simulink model "Matlab_ReadUART"  (R2022b)
settings: Solver=FixedStepAuto  StartTime=0.0  StopTime=inf  FixedStep=0.02  RelTol=1e-3
undefined symbols (not defined in the file): LF
libraries: instrumentseriallib x3, dsparch4 x2, etargetslib x2, dspstat3 x2, simulink_extras x2, aerolibatmos2 x1
settings Model: Creator=tanda  LastModifiedBy=Tan-Dat Le

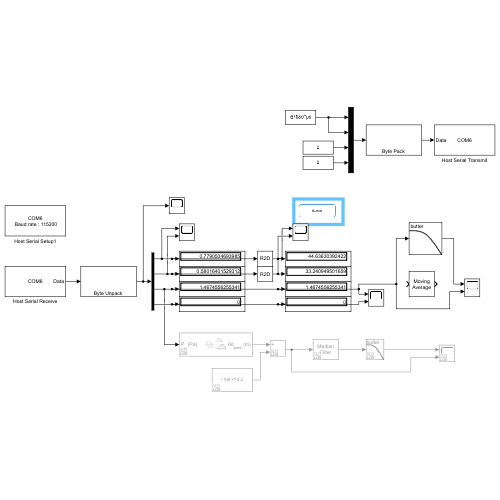
[thumbnail: Simulink's stored preview of the top-level diagram]
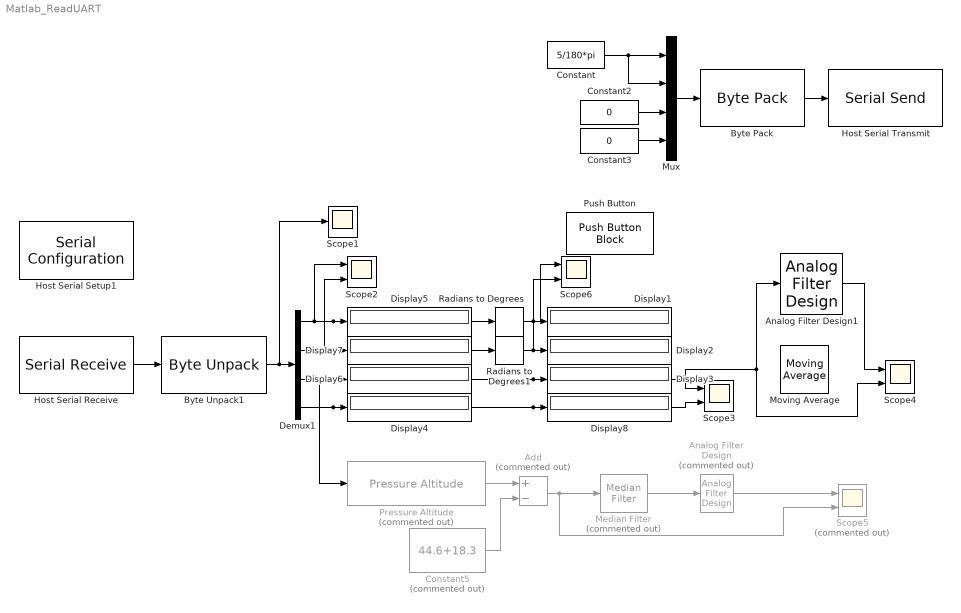
== system Matlab_ReadUART ==
  Add : Sum  Commented=on  Inputs=+-
  Analog Filter Design : dsparch4/Analog Filter Design  Commented=on  method=Butterworth  filttype=Lowpass  N=1  Wlo=0.6  Whi=80  Rp=2  Rs=40
  Analog Filter Design1 : dsparch4/Analog Filter Design  method=Butterworth  filttype=Lowpass  N=1  Wlo=2*pi*0.5  Whi=80  Rp=2  Rs=40
  Byte Pack : etargetslib/Byte Pack  datatypes={'double'}  byteAlign=8
  Byte Unpack1 : etargetslib/Byte Unpack  dimensions={[4]}  datatypes={'double'}  byteAlign=1
      settings: LibrarySourceBlock=embeddedtargetslib/Host Communication/Byte Unpack
  Constant : Constant  Value=5/180*pi
  Constant2 : Constant  Value=0
  Constant3 : Constant  Value=0
  Constant5 : Constant  Commented=on  Value=44.6+18.3
  Demux1 : Demux
  Display{1..8} (8 alike) : Display
  Host Serial Receive : instrumentseriallib/Serial Receive  PortSel=COM6  Port=COM6  ComPort=COM6  DataType=uint8  SaveDataType=uint8  ToggleHeader=on  Header=''  ToggleTerminator=on  Terminator=Custom terminator  CustomTerminator='E'  InputFormat=Row major  ToggleDataSize=on  DataSize=32  EnableBlockingMode=on  ActionDataUnavailable=Output last received value  ActionWhenDataUnavailable=Output last received value  CustomValue=0  SampleTime=-1  SimulateUsing=Interpreted execution  BlockInModel=on  aMode=5
      settings: LibrarySourceBlock=mcblib/Protection and Diagnostics/Host Serial Receive
  Host Serial Setup1 : instrumentseriallib/Serial Configuration  Priority=-99  PortSel=COM6  Port=COM6  ComPort=COM6  BaudRate=115200  DataBits=8  Parity=none  StopBits=1  ByteOrder=little-endian  FlowControl=none  Timeout=1.0  SimulateUsing=Interpreted execution  BlockInModel=on  aMode=5
      settings: LibrarySourceBlock=mcblib/Protection and Diagnostics/Host Serial Setup
  Host Serial Transmit : instrumentseriallib/Serial Send  PortSel=COM6  Port=COM6  ComPort=COM6  Header='S'  Terminator=LF ('\n')  CustomTerminator=''  EnableBlockingMode=off  SimulateUsing=Interpreted execution  BlockInModel=on  aMode=5
      settings: LibrarySourceBlock=mcblib/Protection and Diagnostics/Host Serial Transmit
  Median Filter : dspstat3/Median Filter  Commented=on  WindowLength=5  SimulateUsing=Code generation
      settings: LibrarySourceBlock=|
      | dspfdesign/Median
      | Filter
  Moving Average : dspstat3/Moving Average  Method=Exponential weighting  ForgettingFactorPort=off  SpecifyWindowLength=off  WindowLength=4  OverlapLength=3  AllowArbitraryInputLength=off  ForgettingFactor=0.9  SimulateUsing=Code generation
  Mux : Mux
  Pressure Altitude : aerolibatmos2/Pressure Altitude  Commented=on  units=Metric (MKS)  action=Warning
  Push Button : PushButtonBlock  OffValue=0.000000
  Radians to Degrees : simulink_extras/Transformations/Radians to Degrees
  Radians to Degrees1 : simulink_extras/Transformations/Radians to Degrees
  Scope1 : Scope
  Scope{2..4,6} (4 alike) : Scope  NumInputPorts=2
  Scope5 : Scope  Commented=on  NumInputPorts=2
  wires:
  Demux1/1 -> Scope2/1, Radians to Degrees/1, Display5/1
  Byte Unpack1/1 -> Demux1/1, Scope1/1
  Host Serial Receive/1 -> Byte Unpack1/1
  Byte Pack/1 -> Host Serial Transmit/1
  Mux/1 -> Byte Pack/1
  Constant/1 -> Mux/2, Mux/1
  Constant2/1 -> Mux/3
  Constant3/1 -> Mux/4
  Radians to Degrees/1 -> Scope6/1, Display1/1
  Demux1/2 -> Scope2/2, Radians to Degrees1/1, Display7/1
  Radians to Degrees1/1 -> Scope6/2, Display2/1
  Demux1/4 -> Scope3/2, Display8/1, Display4/1
  Pressure Altitude/1 -> Add/1
  Constant5/1 -> Add/2
  Median Filter/1 -> Analog Filter Design/1
  Add/1 -> Scope5/2, Median Filter/1
  Analog Filter Design/1 -> Scope5/1
  Demux1/3 -> Pressure Altitude/1, Scope3/1, Scope4/2, Analog Filter Design1/1, Display3/1, Display6/1
  Analog Filter Design1/1 -> Scope4/1
